simulink model "controller1_ss"  (R2020a)
settings: Solver=FixedStepAuto  StartTime=0.0  StopTime=22  FixedStep=options.dt  RelTol=1e-3
undefined symbols (not defined in the file or in its folder): A1, B1, C1, den1, num1, options
libraries: simulink x2
settings Model: Creator=kekatos  LastModifiedBy=kekatos
settings DataIOCC: DSMLogging=off  ReturnWorkspaceOutputs=off

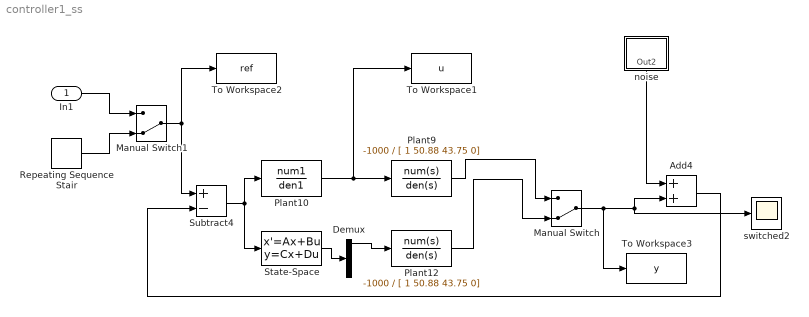
== system controller1_ss ==
  In1 : Inport
  Add4 : Sum
  Demux : Demux
  Manual Switch : ManualSwitch  CurrentSetting=0
  Manual Switch1 : ManualSwitch  CurrentSetting=0
  Plant10 : TransferFcn  Numerator=num1  Denominator=den1
  Plant12 : TransferFcn  Numerator=-1000  Denominator=[ 1 50.88 43.75 0]
  Plant9 : TransferFcn  Numerator=-1000  Denominator=[ 1 50.88 43.75 0]
  Repeating Sequence Stair : simulink/Sources/Repeating Sequence Stair  OutValues=[1 2].'  tsamp=25  OutMin=[]  OutMax=[]  OutDataTypeStr=double  OutputDataTypeScalingMode=double  OutDataType=fixdt(0,8)  ConRadixGroup=Best Precision: Vector-wise  OutScaling=2^-12
  State-Space : StateSpace  A=A1  B=B1  C=[C1;eye(3)]  D=[0;0;0;0]  InitialCondition=0
  Subtract4 : Sum  Inputs=+-
  To Workspace1 : ToWorkspace  VariableName=u  SaveFormat=Structure With Time  SampleTime=options.dt
  To Workspace2 : ToWorkspace  VariableName=ref  SaveFormat=Structure With Time  SampleTime=options.dt
  To Workspace3 : ToWorkspace  VariableName=y  SaveFormat=Structure With Time  SampleTime=options.dt
  noise : Subsystem
  switched2 : Scope
  wires:
  Manual Switch/1 -> To Workspace3/1, switched2/1, Add4/2
  Plant9/1 -> Manual Switch/1
  Plant10/1 -> To Workspace1/1, Plant9/1
  Add4/1 -> Subtract4/2
  Subtract4/1 -> State-Space/1, Plant10/1
  Plant12/1 -> Manual Switch/2
  noise/1(Out2) -> Add4/1
  In1/1 -> Manual Switch1/1
  Repeating Sequence Stair/1 -> Manual Switch1/2
  Manual Switch1/1 -> Subtract4/1, To Workspace2/1
  State-Space/1 -> Demux/1
  Demux/1 -> Plant12/1

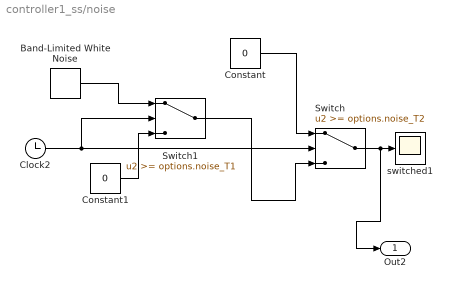
== system controller1_ss/noise ==
  Band-Limited White Noise : simulink/Sources/Band-Limited White Noise  Cov=[0.0001]  Ts=options.dt  seed=[23341]
  Clock2 : Clock
  Constant : Constant  Value=0
  Constant1 : Constant  Value=0
  Switch : Switch  Threshold=options.noise_T2
  Switch1 : Switch  Threshold=options.noise_T1
  switched1 : Scope
  Out2 : Outport
  wires:
  Clock2/1 -> Switch1/2, Switch/2
  Constant/1 -> Switch/1
  Constant1/1 -> Switch1/3
  Band-Limited White Noise/1 -> Switch1/1
  Switch/1 -> Out2/1, switched1/1
  Switch1/1 -> Switch/3
